simulink model "static_mile3"  (R2024b)
settings: Solver=VariableStepAuto  StartTime=0.0  StopTime=5  RelTol=1e-3
undefined symbols (not defined in the file): getTurboIOIndices
libraries: commcnvcod2 x6, commsink2 x4, commdigbbndam3 x4, commdigbbndpm3 x2, commchan3 x1, commrandsrc3 x1
settings Model: Creator=root  LastModifiedBy=root

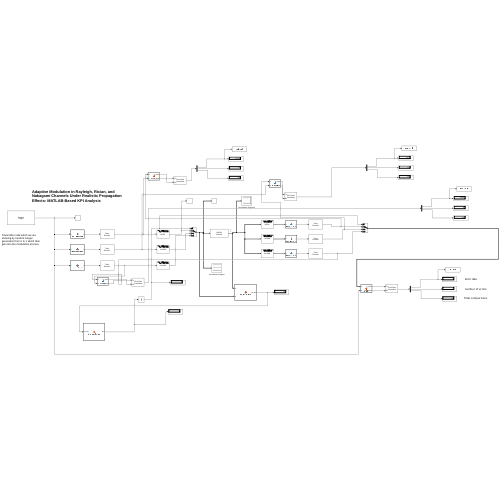
[thumbnail: Simulink's stored preview of the top-level diagram]
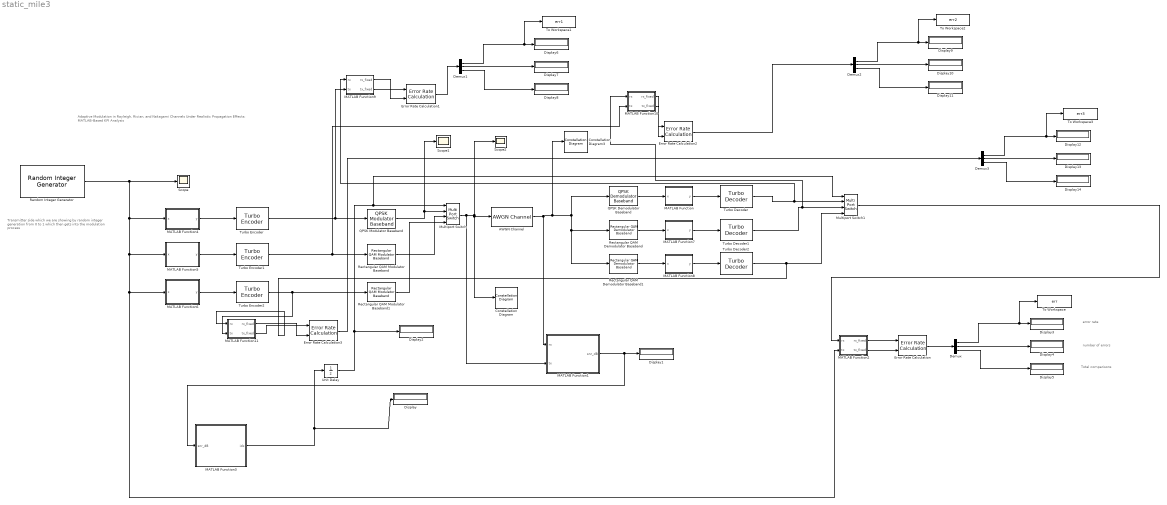
== system static_mile3 ==
  note: Total comparisons
  note: number of errors
  note: Adaptive Modulation in Rayleigh, Rician, and Nakagami Channels Under Realistic Propagation Effects: MATLAB-Based KPI Analysis
  note: error rate
  note: Transmitter side which we are showing by random integer generation from 0 to 1 which then gets into the modulation process
  AWGN Channel : commchan3/AWGN Channel  LegacyMode=off  NoiseMethod="Signal to noise ratio  (SNR)"  noiseMode="Signal to noise ratio  (SNR)"  EbNo=10  EsNo=10  SNR=100  BitsPerSymbol=1  SignalPower=1  SamplesPerSymbol=1  SymbolPeriod=1  VarianceSource=Parameter  Variance=1  RandomStream=Global stream  Seed=67  SimulateUsing=Code generation
  Constellation Diagram : ConstellationDiagram  WindowPosition=[216.000000,65.000000,1440.000000,700.000000,]  Visible=on  ScopeFrameLocation=window
  Constellation Diagram3 : ConstellationDiagram  WindowPosition=[116.000000,65.000000,1440.000000,701.000000,]  Visible=on  ScopeFrameLocation=window
  Demux{,1..3} (4 alike) : Demux  Outputs=3
  Display{,1..14} (15 alike) : Display
  Error Rate Calculation{,1..3} (4 alike) : commsink2/Error Rate Calculation  N=0  st_delay=0  cp_mode=Entire frame  subframe=[]  PMode=Port  WsName=ErrorVec  RsMode2=off  stop=off  numErr=100  maxBits=1e6
      settings: LibrarySourceBlock=|
      | commhdlsink/Error Rate
      | Calculation
  MATLAB Function : MATLAB Function  TreatAsAtomicUnit=on
  MATLAB Function1 : MATLAB Function  TreatAsAtomicUnit=on
  MATLAB Function10 : MATLAB Function  TreatAsAtomicUnit=on
  MATLAB Function11 : MATLAB Function  TreatAsAtomicUnit=on
  MATLAB Function2 : MATLAB Function  TreatAsAtomicUnit=on
  MATLAB Function3 : MATLAB Function  TreatAsAtomicUnit=on
  MATLAB Function4 : MATLAB Function  TreatAsAtomicUnit=on
  MATLAB Function5 : MATLAB Function  TreatAsAtomicUnit=on
  MATLAB Function6 : MATLAB Function  TreatAsAtomicUnit=on
  MATLAB Function7 : MATLAB Function  TreatAsAtomicUnit=on
  MATLAB Function8 : MATLAB Function  TreatAsAtomicUnit=on
  MATLAB Function9 : MATLAB Function  TreatAsAtomicUnit=on
  Multiport Switch : MultiPortSwitch  DataPortOrder=Zero-based contiguous  zeroidx=on  AllowDiffInputSizes=on  SaturateOnIntegerOverflow=off  InputSameDT=off
  Multiport Switch1 : MultiPortSwitch  DataPortOrder=Zero-based contiguous  zeroidx=on  OutDataTypeStr=double  AllowDiffInputSizes=on  SaturateOnIntegerOverflow=off  InputSameDT=off
  QPSK Demodulator Baseband : commdigbbndpm3/QPSK Demodulator Baseband  OutType=Bit  DecType=Hard decision  VarSource=Dialog  Variance=1  Dec=Gray  Ph=pi/4  outDtype1=Inherit via internal rule  outDtype2=Inherit via internal rule  derotateFactorWordLen=16  derotateFactorDataTypeStr=Inherit: Same word length as input  derotateFactorLastDataTypeStr=Inherit: Same word length as input
  QPSK Modulator Baseband : commdigbbndpm3/QPSK Modulator Baseband  InType=Bit  Enc=Gray  Ph=pi/4  outDtype=Inherit via back propagation  outWordLen=16  outUDDataType=sfix(16)  outFracLenMode=Best precision  outFracLen=15  outDataTypeStr=Inherit: Inherit via back propagation  outLastDataTypeStr=Inherit: Inherit via back propagation
  Random Integer Generator : commrandsrc3/Random Integer Generator  SetSize=2  SeedSource=Auto  Seed=0  SampleTime=2  SamplesPerFrame=18000  OutputDataType=double  SimulateUsing=Interpreted execution
  Rectangular QAM Demodulator Baseband : commdigbbndam3/Rectangular QAM Demodulator Baseband  M=16  OutType=Bit  DecType=Hard decision  VarSource=Dialog  Variance=1  Dec=Gray  Mapping=[0:15]  PowType=Min. distance between symbols  MinDist=2  AvgPow=1  PeakPow=1  Ph=0  outDtype1=Inherit via internal rule  outDtype2=Inherit via internal rule  derotateFactorWordLen=16  derotateFactorDataTypeStr=Inherit: Same word length as input  derotateFactorLastDataTypeStr=Inherit: Same word length as input  denormFactorWordLen=16  denormFactorDataTypeStr=Inherit: Same word length as input  denormFactorLastDataTypeStr=Inherit: Same word length as input  prodOutWordLen=32  prodOutOverflowMode=Wrap  prodOutRoundingMode=Floor  prodOutOvFlMode=off  prodOutOvFlModeLastStrValue=off  sumWordLen=32
      settings: LibrarySourceBlock=|
      | commhdldigbbndam/Rectangular QAM
      | Demodulator
      | Baseband
  Rectangular QAM Demodulator Baseband1 : commdigbbndam3/Rectangular QAM Demodulator Baseband  M=64  OutType=Bit  DecType=Hard decision  VarSource=Dialog  Variance=1  Dec=Gray  Mapping=[0:15]  PowType=Min. distance between symbols  MinDist=2  AvgPow=1  PeakPow=1  Ph=0  outDtype1=Inherit via internal rule  outDtype2=Inherit via internal rule  derotateFactorWordLen=16  derotateFactorDataTypeStr=Inherit: Same word length as input  derotateFactorLastDataTypeStr=Inherit: Same word length as input  denormFactorWordLen=16  denormFactorDataTypeStr=Inherit: Same word length as input  denormFactorLastDataTypeStr=Inherit: Same word length as input  prodOutWordLen=32  prodOutOverflowMode=Wrap  prodOutRoundingMode=Floor  prodOutOvFlMode=off  prodOutOvFlModeLastStrValue=off  sumWordLen=32
      settings: LibrarySourceBlock=|
      | commhdldigbbndam/Rectangular QAM
      | Demodulator
      | Baseband
  Rectangular QAM Modulator Baseband : commdigbbndam3/Rectangular QAM Modulator Baseband  M=16  InType=Bit  Enc=Gray  Mapping=[0:15]  PowType=Min. distance between symbols  MinDist=2  AvgPow=1  PeakPow=1  Ph=0  outDtype=Inherit via back propagation  outWordLen=16  outUDDataType=sfix(16)  outFracLenMode=Best precision  outFracLen=15  outDataTypeStr=Inherit: Inherit via back propagation  outLastDataTypeStr=Inherit: Inherit via back propagation
  Rectangular QAM Modulator Baseband1 : commdigbbndam3/Rectangular QAM Modulator Baseband  M=64  InType=Bit  Enc=Gray  Mapping=[0:15]  PowType=Min. distance between symbols  MinDist=2  AvgPow=1  PeakPow=1  Ph=0  outDtype=Inherit via back propagation  outWordLen=16  outUDDataType=sfix(16)  outFracLenMode=Best precision  outFracLen=15  outDataTypeStr=Inherit: Inherit via back propagation  outLastDataTypeStr=Inherit: Inherit via back propagation
  Scope : Scope
  Scope1 : Scope
  Scope2 : Scope
  To Workspace : ToWorkspace  VariableName=err  SampleTime=-1
  To Workspace1 : ToWorkspace  VariableName=err1  SampleTime=-1
  To Workspace2 : ToWorkspace  VariableName=err2  SampleTime=-1
  To Workspace3 : ToWorkspace  VariableName=err3  SampleTime=-1
  Turbo Decoder : commcnvcod2/Turbo Decoder  TrellisStructure=poly2trellis( 4, [ 13, 15 ], 13 )  InterleaverIndicesSource=Property  InterleaverIndices=(64:-1:1).'  InputIndicesSource=Auto  InputIndices=getTurboIOIndices( 64, 2, 3 )  Algorithm=True APP  NumScalingBits=3  NumIterations=25  SimulateUsing=Interpreted execution
  Turbo Decoder1 : commcnvcod2/Turbo Decoder  TrellisStructure=poly2trellis( 4, [ 13, 15 ], 13 )  InterleaverIndicesSource=Property  InterleaverIndices=(64:-1:1).'  InputIndicesSource=Auto  InputIndices=getTurboIOIndices( 64, 2, 3 )  Algorithm=True APP  NumScalingBits=3  NumIterations=25  SimulateUsing=Interpreted execution
  Turbo Decoder2 : commcnvcod2/Turbo Decoder  TrellisStructure=poly2trellis( 4, [ 13, 15 ], 13 )  InterleaverIndicesSource=Property  InterleaverIndices=(64:-1:1).'  InputIndicesSource=Auto  InputIndices=getTurboIOIndices( 64, 2, 3 )  Algorithm=True APP  NumScalingBits=3  NumIterations=25  SimulateUsing=Interpreted execution
  Turbo Encoder : commcnvcod2/Turbo Encoder  TrellisStructure=poly2trellis( 4, [ 13, 15 ], 13 )  InterleaverIndicesSource=Property  InterleaverIndices=(64:-1:1).'  OutputIndicesSource=Auto  OutputIndices=getTurboIOIndices( 64, 2, 3 )  SimulateUsing=Interpreted execution
  Turbo Encoder1 : commcnvcod2/Turbo Encoder  TrellisStructure=poly2trellis( 4, [ 13, 15 ], 13 )  InterleaverIndicesSource=Property  InterleaverIndices=(64:-1:1).'  OutputIndicesSource=Auto  OutputIndices=getTurboIOIndices( 64, 2, 3 )  SimulateUsing=Interpreted execution
  Turbo Encoder2 : commcnvcod2/Turbo Encoder  TrellisStructure=poly2trellis( 4, [ 13, 15 ], 13 )  InterleaverIndicesSource=Property  InterleaverIndices=(64:-1:1).'  OutputIndicesSource=Auto  OutputIndices=getTurboIOIndices( 64, 2, 3 )  SimulateUsing=Interpreted execution
  Unit Delay : UnitDelay  InitialCondition=1  SampleTime=2  HasFrameUpgradeWarning=on
  wires:
  Turbo Encoder2/1 -> Rectangular QAM Modulator Baseband1/1, MATLAB Function11/2(tx)
  MATLAB Function8/1(y) -> Turbo Decoder2/1
  MATLAB Function/1(y) -> Turbo Decoder/1
  Turbo Encoder1/1 -> MATLAB Function10/2(tx), Rectangular QAM Modulator Baseband/1
  MATLAB Function7/1(y) -> Turbo Decoder1/1
  Rectangular QAM Modulator Baseband1/1 -> Multiport Switch/4
  MATLAB Function6/1(y) -> Turbo Encoder2/1
  Rectangular QAM Demodulator Baseband1/1 -> MATLAB Function8/1(x)
  MATLAB Function2/1(rx_fixed) -> Error Rate Calculation/1
  MATLAB Function2/2(tx_fixed) -> Error Rate Calculation/2
  Turbo Decoder1/1 -> MATLAB Function10/1(rx), Multiport Switch1/3
  Turbo Encoder/1 -> MATLAB Function9/2(tx), QPSK Modulator Baseband/1
  Rectangular QAM Demodulator Baseband/1 -> MATLAB Function7/1(x)
  QPSK Modulator Baseband/1 -> Multiport Switch/2, Scope1/1
  Error Rate Calculation/1 -> Demux/1
  Random Integer Generator/1 -> Scope/1, MATLAB Function2/2(tx), MATLAB Function6/1(x), MATLAB Function5/1(x), MATLAB Function4/1(x)
  Demux/1 -> To Workspace/1, Display3/1
  Demux/3 -> Display5/1
  Multiport Switch/1 -> MATLAB Function1/2(tx), Constellation Diagram/1, AWGN Channel/1, Scope2/1
  Multiport Switch1/1 -> MATLAB Function2/1(rx)
  MATLAB Function4/1(y) -> Turbo Encoder/1
  Demux/2 -> Display4/1
  Turbo Decoder/1 -> MATLAB Function9/1(rx), Multiport Switch1/2
  Unit Delay/1 -> Multiport Switch1/1, Multiport Switch/1, Display2/1
  Rectangular QAM Modulator Baseband/1 -> Multiport Switch/3
  QPSK Demodulator Baseband/1 -> MATLAB Function/1(x)
  AWGN Channel/1 -> Constellation Diagram3/1, Rectangular QAM Demodulator Baseband1/1, Rectangular QAM Demodulator Baseband/1, QPSK Demodulator Baseband/1, MATLAB Function1/1(rx)
  Turbo Decoder2/1 -> MATLAB Function11/1(rx), Multiport Switch1/4
  MATLAB Function1/1(snr_dB) -> Display1/1, MATLAB Function3/1(snr_dB)
  MATLAB Function3/1(idx) -> Unit Delay/1, Display/1
  MATLAB Function5/1(y) -> Turbo Encoder1/1
  Demux1/1 -> To Workspace1/1, Display6/1
  Demux1/3 -> Display8/1
  Demux1/2 -> Display7/1
  Error Rate Calculation1/1 -> Demux1/1
  Demux2/1 -> To Workspace2/1, Display9/1
  Demux2/3 -> Display11/1
  Demux2/2 -> Display10/1
  Error Rate Calculation2/1 -> Demux2/1
  Demux3/1 -> To Workspace3/1, Display12/1
  Demux3/3 -> Display14/1
  Demux3/2 -> Display13/1
  Error Rate Calculation3/1 -> Demux3/1
  MATLAB Function9/1(rx_fixed) -> Error Rate Calculation1/2
  MATLAB Function9/2(tx_fixed) -> Error Rate Calculation1/1
  MATLAB Function10/1(rx_fixed) -> Error Rate Calculation2/2
  MATLAB Function10/2(tx_fixed) -> Error Rate Calculation2/1
  MATLAB Function11/2(tx_fixed) -> Error Rate Calculation3/1
  MATLAB Function11/1(rx_fixed) -> Error Rate Calculation3/2

== matlab function static_mile3/MATLAB Function ==
  data: x input; y output
function y = my_wrapper(x)
%#codegen
y = zeros(204, 1);  % match encoder output length
N = min(length(x), 204);
y(1:N) = x(1:N);

== matlab function static_mile3/MATLAB Function2 ==
  data: rx input; rx_fixed output; tx input; tx_fixed output
function [rx_fixed, tx_fixed] = fixTo64(rx, tx)
%#codegen
% Ensure both outputs are always exactly 64×1

  % Pre‐allocate 64×1 outputs
  rx_fixed = zeros(64,1);
  tx_fixed = zeros(64,1);

  % How many samples we really have
  Lr = numel(rx);
  Lt = numel(tx);

  % Truncate or pad rx
  if Lr >= 64
    rx_fixed = rx(1:64);
  else
    rx_fixed(1:Lr) = rx;
  end

  % Truncate or pad tx
  if Lt >= 64
    tx_fixed = tx(1:64);
  else
    tx_fixed(1:Lt) = tx;
  end
end

== matlab function static_mile3/MATLAB Function3 ==
  data: snr_dB input; idx output
function idx = amc_controller(snr_dB)
%#codegen

% Define SNR thresholds for modulation + coding selection
if snr_dB < 7
    idx = 0;  % QPSK
elseif snr_dB < 15
    idx = 1;  % 16-QAM
else
    idx = 2;  % 64-QAM
end

== matlab function static_mile3/MATLAB Function4 ==
  data: x input; y output
function y = truncatePad64(x)
%#codegen
N = length(x);
fixedLen = 64;

% Allocate a [64 x 1] output
y = zeros(fixedLen,1);

% If input has more than 64 bits, truncate
if N >= fixedLen
    y(1:fixedLen) = x(1:fixedLen);
else
    % If input is shorter, copy + zero pad
    y(1:N) = x(1:N);
    % The rest remain zeros
end

== matlab function static_mile3/MATLAB Function5 ==
  data: x input; y output
function y = truncatePad64(x)
%#codegen
N = length(x);
fixedLen = 64;

% Allocate a [64 x 1] output
y = zeros(fixedLen,1);

% If input has more than 64 bits, truncate
if N >= fixedLen
    y(1:fixedLen) = x(1:fixedLen);
else
    % If input is shorter, copy + zero pad
    y(1:N) = x(1:N);
    % The rest remain zeros
end

== matlab function static_mile3/MATLAB Function6 ==
  data: x input; y output
function y = truncatePad64(x)
%#codegen
N = length(x);
fixedLen = 64;

% Allocate a [64 x 1] output
y = zeros(fixedLen,1);

% If input has more than 64 bits, truncate
if N >= fixedLen
    y(1:fixedLen) = x(1:fixedLen);
else
    % If input is shorter, copy + zero pad
    y(1:N) = x(1:N);
    % The rest remain zeros
end

== matlab function static_mile3/MATLAB Function7 ==
  data: x input; y output
function y = my_wrapper(x)
%#codegen
y = zeros(204, 1);  % match encoder output length
N = min(length(x), 204);
y(1:N) = x(1:N);

== matlab function static_mile3/MATLAB Function8 ==
  data: x input; y output
function y = my_wrapper(x)
%#codegen
y = zeros(204, 1);  % match encoder output length
N = min(length(x), 204);
y(1:N) = x(1:N);

== matlab function static_mile3/MATLAB Function9 ==
  data: rx input; rx_fixed output; tx input; tx_fixed output
function [rx_fixed, tx_fixed] = fixTo64(rx, tx)
%#codegen
% Ensure both outputs are always exactly 64×1

  % Pre‐allocate 64×1 outputs
  rx_fixed = zeros(64,1);
  tx_fixed = zeros(64,1);

  % How many samples we really have
  Lr = numel(rx);
  Lt = numel(tx);

  % Truncate or pad rx
  if Lr >= 64
    rx_fixed = rx(1:64);
  else
    rx_fixed(1:Lr) = rx;
  end

  % Truncate or pad tx
  if Lt >= 64
    tx_fixed = tx(1:64);
  else
    tx_fixed(1:Lt) = tx;
  end
end

== matlab function static_mile3/MATLAB Function10 ==
  data: rx input; rx_fixed output; tx input; tx_fixed output
function [rx_fixed, tx_fixed] = fixTo64(rx, tx)
%#codegen
% Ensure both outputs are always exactly 64×1

  % Pre‐allocate 64×1 outputs
  rx_fixed = zeros(64,1);
  tx_fixed = zeros(64,1);

  % How many samples we really have
  Lr = numel(rx);
  Lt = numel(tx);

  % Truncate or pad rx
  if Lr >= 64
    rx_fixed = rx(1:64);
  else
    rx_fixed(1:Lr) = rx;
  end

  % Truncate or pad tx
  if Lt >= 64
    tx_fixed = tx(1:64);
  else
    tx_fixed(1:Lt) = tx;
  end
end

== matlab function static_mile3/MATLAB Function1 ==
  data: rx input; snr_dB output; tx input
function snr_dB = snr_estimator(rx, tx)
%#codegen
    noise     = rx - tx;          % estimation of the noise
    P_noise   = norm(noise)^2;    % total noise energy
    P_signal  = norm(tx)^2;       % total signal energy
    snr_dB    = 10 * log10(P_signal / P_noise);
end

== matlab function static_mile3/MATLAB Function11 ==
  data: rx input; rx_fixed output; tx input; tx_fixed output
function [rx_fixed, tx_fixed] = fixTo64(rx, tx)
%#codegen
% Ensure both outputs are always exactly 64×1

  % Pre‐allocate 64×1 outputs
  rx_fixed = zeros(64,1);
  tx_fixed = zeros(64,1);

  % How many samples we really have
  Lr = numel(rx);
  Lt = numel(tx);

  % Truncate or pad rx
  if Lr >= 64
    rx_fixed = rx(1:64);
  else
    rx_fixed(1:Lr) = rx;
  end

  % Truncate or pad tx
  if Lt >= 64
    tx_fixed = tx(1:64);
  else
    tx_fixed(1:Lt) = tx;
  end
end
